simulink library "clutchMotorLib"  (R2018a)
settings: Solver=VariableStepAuto  StartTime=0.0  StopTime=10.0  RelTol=1e-3
settings Model: Creator=SIMONE  LastModifiedBy=SIMONE

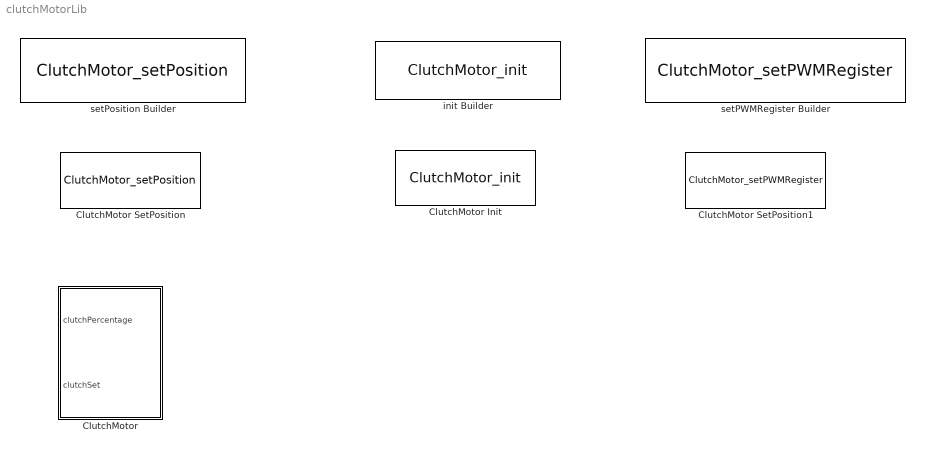
== system clutchMotorLib ==
  ClutchMotor : Subsystem
  ClutchMotor Init : S-Function  FunctionName=ClutchMotor_init  SFunctionDeploymentMode=off  EnableBusSupport=off
  ClutchMotor SetPosition : S-Function  FunctionName=ClutchMotor_setPosition  SFunctionDeploymentMode=off  EnableBusSupport=off
  ClutchMotor SetPosition1 : S-Function  FunctionName=ClutchMotor_setPWMRegister  SFunctionDeploymentMode=off  EnableBusSupport=off
  init Builder : S-Function  InitFcn=try, set_param(gcb,'FunctionName','ClutchMotor_init'), end  FunctionName=ClutchMotor_init  SFunctionModules=ClutchMotor_init_wrapper ClutchMotor_setPosition_wrapper  SFunctionDeploymentMode=off  EnableBusSupport=off  mask(S-Function Builder){}
      mask help: Simulink:masks:SFunctionBuilder_MD
      mask init:
      | val = [[.9  0.75 0.75 1 1 .9 .9 1]',[1 1 0.75 0.75 .9 .9 1 .9]'];try , sys = get_param(gcb,'SfunBuilderFcnName');if isempty(sys), sys = get_param(gcb,'FunctionName'); end,catch, sys = get_param(gcb,'FunctionName'); end
      settings: CopyFcn=set_param(gcbh,'LinkStatus','none')  PreSaveFcn=try, set_param(gcb,'FunctionName','ClutchMotor_init'), end  OpenFcn=sfunctionwizard(gcbh)
      mask Display:
      | plot(val(:,1),val(:,2))
      | disp(sys)
  setPWMRegister Builder : S-Function  InitFcn=try, set_param(gcb,'FunctionName','ClutchMotor_setPWMRegister'), end  FunctionName=ClutchMotor_setPWMRegister  SFunctionModules=ClutchMotor_setPWMRegister_wrapper  SFunctionDeploymentMode=off  EnableBusSupport=off  mask(S-Function Builder){}
      mask help: Simulink:masks:SFunctionBuilder_MD
      mask init: same as clutchMotorLib/init Builder
      settings: CopyFcn=set_param(gcbh,'LinkStatus','none')  PreSaveFcn=try, set_param(gcb,'FunctionName','ClutchMotor_setPWMRegister'), end  OpenFcn=sfunctionwizard(gcbh)
      mask Display: plot(val(:,1),val(:,2)),disp(sys), port_label('input',1,'pwmValue')
  setPosition Builder : S-Function  InitFcn=try, set_param(gcb,'FunctionName','ClutchMotor_setPosition'), end  FunctionName=ClutchMotor_setPosition  SFunctionModules=ClutchMotor_setPosition_wrapper  SFunctionDeploymentMode=off  EnableBusSupport=off  mask(S-Function Builder){}
      mask help: Simulink:masks:SFunctionBuilder_MD
      mask init: same as clutchMotorLib/init Builder
      settings: CopyFcn=set_param(gcbh,'LinkStatus','none')  PreSaveFcn=try, set_param(gcb,'FunctionName','ClutchMotor_setPosition'), end  OpenFcn=sfunctionwizard(gcbh)
      mask Display: plot(val(:,1),val(:,2)),disp(sys), port_label('input',1,'percentage')

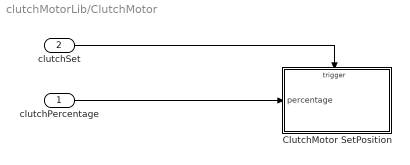
== system clutchMotorLib/ClutchMotor ==
  clutchPercentage : Inport
  clutchSet : Inport  Port=2
  "ClutchMotor SetPosition " : Subsystem  TreatAsAtomicUnit=on
  wires:
  clutchSet/1 -> "ClutchMotor SetPosition "/Trigger
  clutchPercentage/1 -> "ClutchMotor SetPosition "/1(percentage)

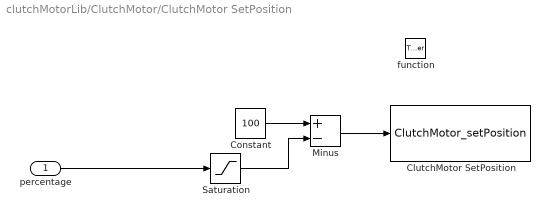
== system clutchMotorLib/ClutchMotor/ClutchMotor SetPosition  ==
  percentage : Inport
  function : TriggerPort  TriggerType=function-call  VariantControl=Variant
  ClutchMotor SetPosition : S-Function  FunctionName=ClutchMotor_setPosition  SFunctionDeploymentMode=off  EnableBusSupport=off
  Constant : Constant  Value=100  OutDataTypeStr=uint8
  Minus : Sum  Inputs=+-
  Saturation : Saturate  UpperLimit=100  LowerLimit=0  ZeroCross=off
  wires:
  Minus/1 -> ClutchMotor SetPosition/1
  Constant/1 -> Minus/1
  Saturation/1 -> Minus/2
  percentage/1 -> Saturation/1
